simulink model "ServoModel_v2"  (R2021b)
settings: Solver=FixedStepAuto  StartTime=0.0  StopTime=Inf  RelTol=1e-3  EnableMultiTasking=on
libraries: simulink x1
settings Model: ExtModeTrigDuration=2  Creator=diego  LastModifiedBy=diego
settings OptimizationCC: EnhancedBackFolding=on  PassReuseOutputArgsAs=Individual arguments  ZeroExternalMemoryAtStartup=off  ZeroInternalMemoryAtStartup=off  MaxStackSize=64  OptimizeBlockOrder=speed  DifferentSizesBufferReuse=on  EfficientTunableParamExpr=on
settings DebuggingCC: ParameterTunabilityLossMsg=error
settings HardwareCC: ProdBitPerInt=16  ProdBitPerPointer=16  ProdBitPerSizeT=16  ProdBitPerPtrDiffT=16  ProdLargestAtomicFloat=None  ProdWordSize=8  ProdHWDeviceType=Atmel->AVR
settings SFSimCC: MATLABDynamicMemAlloc=off
settings RTWCC: Description=Embedded Coder  SystemTargetFile=ert.tlc  HardwareBoard=Arduino Uno  TemplateMakefile=ert_default_tmf  Toolchain=Arduino AVR  BuildConfiguration=Faster Runs
settings CodeAppCC: ForceParamTrailComments=on  IgnoreCustomStorageClasses=off  OperatorAnnotations=on  SimulinkDataObjDesc=on  SFDataObjDesc=on  InsertBlockDesc=on
settings ERTTargetCC: SupportContinuousTime=on  SupportVariableSizeSignals=on  ExtModeTransport=3  ExtModeStaticAlloc=on  ExtModeStaticAllocSize=250  ExtModeMexFile=ext_xcp  ExtModeIntrfLevel=Level2 - Open

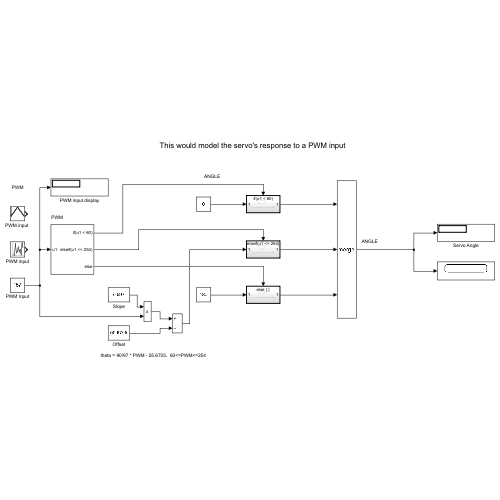
[thumbnail: Simulink's stored preview of the top-level diagram]
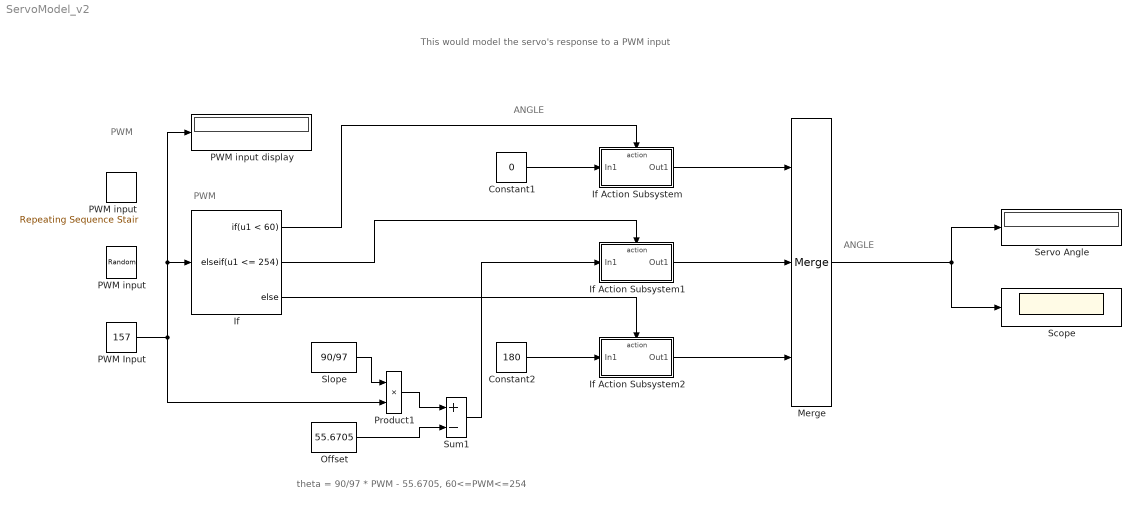
== system ServoModel_v2 ==
  note: This would model the servo's response to a PWM input
  note: theta = 90/97 * PWM - 55.6705, 60<=PWM<=254
  note: PWM
  note: PWM
  note: ANGLE
  note: ANGLE
  Constant1 : Constant  Value=0
  Constant2 : Constant  Value=180
  If : If  IfExpression=u1 < 60  ElseIfExpressions=u1 <= 254
  If Action Subsystem : Subsystem  TreatAsAtomicUnit=on
  If Action Subsystem1 : Subsystem  TreatAsAtomicUnit=on
  If Action Subsystem2 : Subsystem  TreatAsAtomicUnit=on
  Merge : Merge  Inputs=3
  Offset : Constant  Value=55.6705
  PWM Input : Constant  Value=157
  PWM input : UniformRandomNumber  Minimum=0  Maximum=255  Seed=66  SampleTime=0.05
  "PWM input " : simulink/Sources/Repeating Sequence Stair  OutValues=[60:255 254:-1:61]  tsamp=5  OutMin=[0]  OutMax=[255]  OutDataTypeStr=uint8  OutputDataTypeScalingMode=uint8  OutDataType=fixdt(0,8)  ConRadixGroup=Best Precision: Vector-wise  OutScaling=2^-12
  PWM input display : Display
  Product1 : Product
  Scope : Scope
  Servo Angle : Display
  Slope : Constant  Value=90/97
  Sum1 : Sum  Inputs=+-
  wires:
  Offset/1 -> Sum1/2
  Product1/1 -> Sum1/1
  Slope/1 -> Product1/1
  If/1 -> If Action Subsystem/Action
  If/2 -> If Action Subsystem1/Action
  If/3 -> If Action Subsystem2/Action
  If Action Subsystem1/1(Out1) -> Merge/2
  If Action Subsystem/1(Out1) -> Merge/1
  If Action Subsystem2/1(Out1) -> Merge/3
  Merge/1 -> Servo Angle/1, Scope/1
  Constant1/1 -> If Action Subsystem/1(In1)
  Constant2/1 -> If Action Subsystem2/1(In1)
  Sum1/1 -> If Action Subsystem1/1(In1)
  PWM Input/1 -> Product1/2, If/1, PWM input display/1

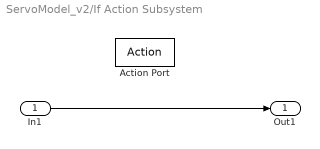
== system ServoModel_v2/If Action Subsystem ==
  In1 : Inport
  Action Port : ActionPort  ActionPortLabel=if(u1 < 60)
  Out1 : Outport
  wires:
  In1/1 -> Out1/1

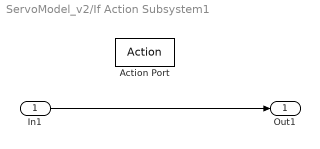
== system ServoModel_v2/If Action Subsystem1 ==
  In1 : Inport
  Action Port : ActionPort  ActionPortLabel=elseif(u1 <= 254)
  Out1 : Outport
  wires:
  In1/1 -> Out1/1

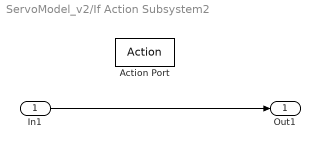
== system ServoModel_v2/If Action Subsystem2 ==
  In1 : Inport
  Action Port : ActionPort  ActionPortLabel=else
  Out1 : Outport
  wires:
  In1/1 -> Out1/1
